simulink model "lab2part1"  (R2018a)
settings: Solver=VariableStepAuto  StartTime=0.0  StopTime=2  RelTol=1e-3
settings Model: Creator=wardzin3  LastModifiedBy=wardzin3

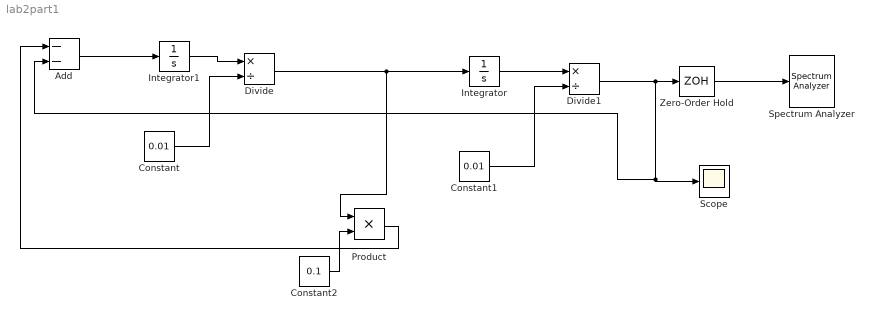
== system lab2part1 ==
  Add : Sum  Inputs=--
  Constant : Constant  Value=0.01
  Constant1 : Constant  Value=0.01
  Constant2 : Constant  Value=0.1
  Divide : Product  Inputs=*/
  Divide1 : Product  Inputs=*/
  Integrator : Integrator  InitialCondition=0.1
  Integrator1 : Integrator  InitialCondition=0.1
  Product : Product
  Scope : Scope
  Spectrum Analyzer : SpectrumAnalyzer
  Zero-Order Hold : ZeroOrderHold  SampleTime=2^(-10)
  wires:
  Integrator1/1 -> Divide/1
  Constant/1 -> Divide/2
  Constant1/1 -> Divide1/2
  Integrator/1 -> Divide1/1
  Divide/1 -> Product/1, Integrator/1
  Constant2/1 -> Product/2
  Zero-Order Hold/1 -> Spectrum Analyzer/1
  Divide1/1 -> Add/2, Scope/1, Zero-Order Hold/1
  Product/1 -> Add/1
  Add/1 -> Integrator1/1
